simulink library "AeroModel"  (R2021b)
settings: Solver=VariableStepAuto  StartTime=0.0  StopTime=10.0  RelTol=1e-3
undefined symbols (not defined in the file or in its folder): b_ft, C_D0, C_Dalpha, C_DdeltaE, C_L0, C_Lalpha, C_Lalphadot, C_lbeta, C_ldeltaA, C_LdeltaE, C_ldeltaR, C_lp, C_Lq, C_lr, C_m0, C_malpha, C_malphadot, C_mdeltaE, C_mq, C_nbeta, C_ndeltaA, C_ndeltaR, C_np, C_nr, C_Ybeta, C_YdeltaA, C_YdeltaR, C_Yp, C_Yr, mean_c_ft, S_ft2
settings Model: Creator=setup  LastModifiedBy=dmgp1

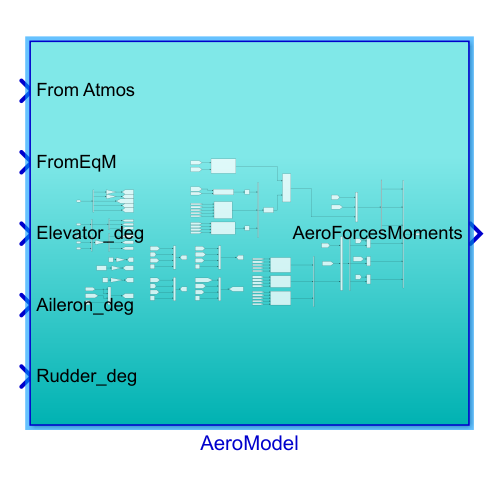
[thumbnail: Simulink's stored preview of the top-level diagram]
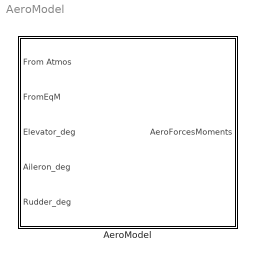
== system AeroModel ==
  AeroModel : Subsystem

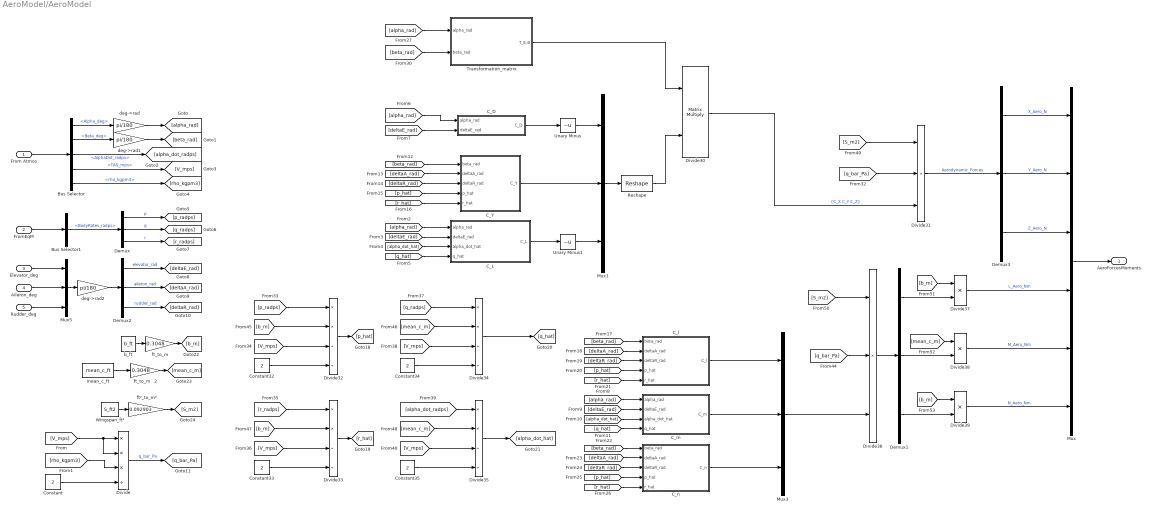
== system AeroModel/AeroModel ==
  From Atmos : Inport
  FromEqM : Inport  Port=2
  Elevator_deg : Inport  Port=3
  Aileron_deg : Inport  Port=4
  Rudder_deg : Inport  Port=5
  Bus Selector : BusSelector  OutputSignals=Alpha_deg,Beta_deg,AlphaDot_radps,TAS_mps,rho_kgpm3
  Bus Selector1 : BusSelector  OutputSignals=BodyRates_radps
  C_D : Subsystem
  C_L : Subsystem
  C_Y : Subsystem
  C_l : Subsystem
  C_m : Subsystem
  C_n : Subsystem
  Constant{,32..35} (5 alike) : Constant  Value=2
  Demux{,1..3} (4 alike) : Demux  Outputs=3
  Divide : Product  Inputs=***/
  Divide30 : Product  Inputs=**  Multiplication=Matrix(*)
  Divide31 : Product  Inputs=***
  Divide{32..35} (4 alike) : Product  Inputs=**//
  Divide36 : Product  Inputs=***
  Divide37 : Product  Inputs=**
  Divide38 : Product  Inputs=**
  Divide39 : Product  Inputs=**
  Mux : Mux  Inputs=6
  Mux1 : Mux  Inputs=3
  Mux3 : Mux  Inputs=3
  Mux5 : Mux  Inputs=3
  Reshape : Reshape  OutputDimensionality=Column vector (2-D)
  Transformation_matrix : Subsystem
  Unary Minus : UnaryMinus
  Unary Minus1 : UnaryMinus
  Wingspan_ft² : Constant  Value=S_ft2
  b_ft : Constant  Value=b_ft
  deg->rad : Gain  Gain=pi/180
  deg->rad1 : Gain  Gain=pi/180
  deg->rad2 : Gain  Gain=pi/180
  ft_to_m : Gain  Gain=0.3048
  ft_to_m   2 : Gain  Gain=0.3048
  ft²_to_m² : Gain  Gain=0.092903
  mean_c_ft : Constant  Value=mean_c_ft
  AeroForcesMoments : Outport
  wires:
  Rudder_deg/1 -> Mux5/3
  Bus Selector/3 -> [alpha_dot_radps]  "<AlphaDot_radps>"
  Bus Selector1/1 -> Demux/1  "<BodyRates_radps>"
  Demux3/3 -> Mux/3  "Z_Aero_N"
  Demux/3 -> [r_radps]  "r"
  Divide37/1 -> Mux/4  "L_Aero_Nm"
  Demux3/2 -> Mux/2  "Y_Aero_N"
  Elevator_deg/1 -> Mux5/1
  Bus Selector/5 -> [rho_kgpm3]  "<rho_kgpm3>"
  Demux/1 -> [p_radps]  "p"
  Aileron_deg/1 -> Mux5/2
  Demux/2 -> [q_radps]  "q"
  From Atmos/1 -> Bus Selector/1
  Demux3/1 -> Mux/1  "X_Aero_N"
  FromEqM/1 -> Bus Selector1/1
  Bus Selector/4 -> [V_mps]  "<TAS_mps>"
  Bus Selector/2 -> deg->rad1/1  "<Beta_deg>"
  Divide38/1 -> Mux/5  "M_Aero_Nm"
  Bus Selector/1 -> deg->rad/1  "<Alpha_deg>"
  Divide39/1 -> Mux/6  "N_Aero_Nm"
  Mux/1 -> AeroForcesMoments/1
  Constant/1 -> Divide/4
  [rho_kgpm3] -> Divide/3
  Demux1/1 -> Divide37/2
  Divide/1 -> [q_bar_Pa]  "q_bar_Pa"
  [b_m] -> Divide33/2
  [q_bar_Pa] -> Divide36/2
  Divide36/1 -> Demux1/1
  [V_mps] -> Divide32/3
  Unary Minus1/1 -> Mux1/3
  b_ft/1 -> ft_to_m/1
  [q_radps] -> Divide34/1
  Divide34/1 -> [q_hat]
  [p_radps] -> Divide32/1
  Demux1/3 -> Divide39/2
  [b_m] -> Divide37/1
  [b_m] -> Divide39/1
  [mean_c_m] -> Divide34/2
  [V_mps] -> Divide33/3
  [mean_c_m] -> Divide38/1
  [b_m] -> Divide32/2
  Demux1/2 -> Divide38/2
  [mean_c_m] -> Divide35/2
  C_m/1(C_m) -> Mux3/2
  [alpha_dot_radps] -> Divide35/1
  [S_m2] -> Divide31/1
  [V_mps] -> Divide/2, Divide/1
  Constant35/1 -> Divide35/4
  ft_to_m/1 -> [b_m]
  Mux1/1 -> Reshape/1
  Constant34/1 -> Divide34/4
  mean_c_ft/1 -> ft_to_m   2/1
  Mux3/1 -> Divide36/3
  C_l/1(C_l) -> Mux3/1
  [V_mps] -> Divide34/3
  [V_mps] -> Divide35/3
  [r_radps] -> Divide33/1
  Divide35/1 -> [alpha_dot_hat]
  C_n/1(C_n) -> Mux3/3
  Constant32/1 -> Divide32/4
  Divide33/1 -> [r_hat]
  Constant33/1 -> Divide33/4
  Divide30/1 -> Divide31/3  "{C_X C_Y C_Z}"
  [q_bar_Pa] -> Divide31/2
  Wingspan_ft²/1 -> ft²_to_m²/1
  [S_m2] -> Divide36/1
  C_D/1(C_D) -> Unary Minus/1
  Reshape/1 -> Divide30/2
  C_L/1(C_L) -> Unary Minus1/1
  ft²_to_m²/1 -> [S_m2]
  ft_to_m   2/1 -> [mean_c_m]
  C_Y/1(C_Y) -> Mux1/2
  Unary Minus/1 -> Mux1/1
  Divide32/1 -> [p_hat]
  deg->rad/1 -> [alpha_rad]
  deg->rad1/1 -> [beta_rad]
  Mux5/1 -> deg->rad2/1
  deg->rad2/1 -> Demux2/1
  Demux2/1 -> [deltaE_rad]  "elevator_rad"
  Demux2/2 -> [deltaA_rad]  "aileron_rad"
  Demux2/3 -> [deltaR_rad]  "rudder_rad"
  [alpha_rad] -> C_D/1(alpha_rad)
  [deltaE_rad] -> C_D/2(deltaE_rad)
  Transformation_matrix/1(T_E,B) -> Divide30/1
  [alpha_rad] -> Transformation_matrix/1(alpha_rad)
  [beta_rad] -> Transformation_matrix/2(beta_rad)
  [beta_rad] -> C_Y/1(beta_rad)
  [deltaA_rad] -> C_Y/2(deltaA_rad)
  [deltaR_rad] -> C_Y/3(deltaR_rad)
  [p_hat] -> C_Y/4(p_hat)
  [r_hat] -> C_Y/5(r_hat)
  [alpha_rad] -> C_L/1(alpha_rad)
  [deltaE_rad] -> C_L/2(deltaE_rad)
  [alpha_dot_hat] -> C_L/3(alpha_dot_hat)
  [q_hat] -> C_L/4(q_hat)
  Divide31/1 -> Demux3/1  "Aerodynamic_Forces"
  [beta_rad] -> C_l/1(beta_rad)
  [deltaA_rad] -> C_l/2(deltaA_rad)
  [deltaR_rad] -> C_l/3(deltaR_rad)
  [p_hat] -> C_l/4(p_hat)
  [r_hat] -> C_l/5(r_hat)
  [alpha_rad] -> C_m/1(alpha_rad)
  [deltaE_rad] -> C_m/2(deltaE_rad)
  [alpha_dot_hat] -> C_m/3(alpha_dot_hat)
  [q_hat] -> C_m/4(q_hat)
  [beta_rad] -> C_n/1(beta_rad)
  [deltaA_rad] -> C_n/2(deltaA_rad)
  [deltaR_rad] -> C_n/3(deltaR_rad)
  [p_hat] -> C_n/4(p_hat)
  [r_hat] -> C_n/5(r_hat)

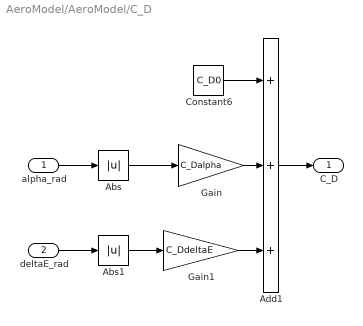
== system AeroModel/AeroModel/C_D ==
  alpha_rad : Inport
  deltaE_rad : Inport  Port=2
  Abs : Abs
  Abs1 : Abs
  Add1 : Sum  Inputs=+++
  Constant6 : Constant  Value=C_D0
  Gain : Gain  Gain=C_Dalpha
  Gain1 : Gain  Gain=C_DdeltaE
  C_D : Outport
  wires:
  Constant6/1 -> Add1/1
  deltaE_rad/1 -> Abs1/1
  Add1/1 -> C_D/1
  Abs/1 -> Gain/1
  Gain/1 -> Add1/2
  alpha_rad/1 -> Abs/1
  Gain1/1 -> Add1/3
  Abs1/1 -> Gain1/1

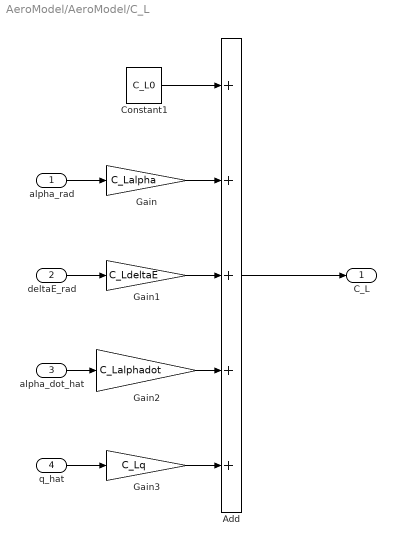
== system AeroModel/AeroModel/C_L ==
  alpha_rad : Inport
  deltaE_rad : Inport  Port=2
  alpha_dot_hat : Inport  Port=3
  q_hat : Inport  Port=4
  Add : Sum  Inputs=+++++
  Constant1 : Constant  Value=C_L0
  Gain : Gain  Gain=C_Lalpha
  Gain1 : Gain  Gain=C_LdeltaE
  Gain2 : Gain  Gain=C_Lalphadot
  Gain3 : Gain  Gain=C_Lq
  C_L : Outport
  wires:
  Gain2/1 -> Add/4
  Add/1 -> C_L/1
  Gain1/1 -> Add/3
  Gain3/1 -> Add/5
  Constant1/1 -> Add/1
  Gain/1 -> Add/2
  alpha_rad/1 -> Gain/1
  deltaE_rad/1 -> Gain1/1
  alpha_dot_hat/1 -> Gain2/1
  q_hat/1 -> Gain3/1

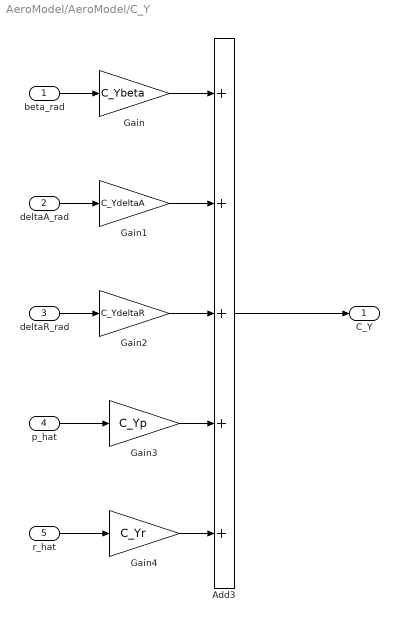
== system AeroModel/AeroModel/C_Y ==
  beta_rad : Inport
  deltaA_rad : Inport  Port=2
  deltaR_rad : Inport  Port=3
  p_hat : Inport  Port=4
  r_hat : Inport  Port=5
  Add3 : Sum  Inputs=+++++
  Gain : Gain  Gain=C_Ybeta
  Gain1 : Gain  Gain=C_YdeltaA
  Gain2 : Gain  Gain=C_YdeltaR
  Gain3 : Gain  Gain=C_Yp
  Gain4 : Gain  Gain=C_Yr
  C_Y : Outport
  wires:
  Add3/1 -> C_Y/1
  Gain1/1 -> Add3/2
  Gain/1 -> Add3/1
  Gain2/1 -> Add3/3
  Gain4/1 -> Add3/5
  Gain3/1 -> Add3/4
  beta_rad/1 -> Gain/1
  deltaA_rad/1 -> Gain1/1
  r_hat/1 -> Gain4/1
  deltaR_rad/1 -> Gain2/1
  p_hat/1 -> Gain3/1

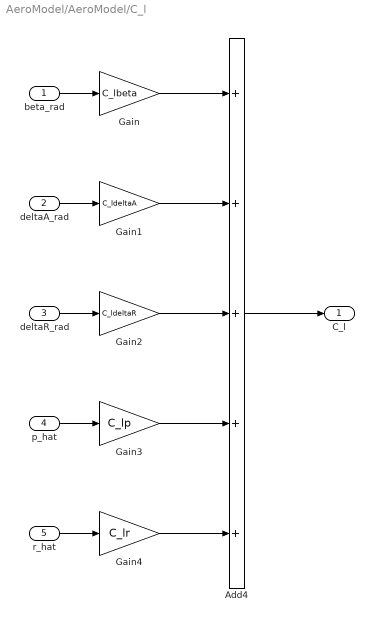
== system AeroModel/AeroModel/C_l ==
  beta_rad : Inport
  deltaA_rad : Inport  Port=2
  deltaR_rad : Inport  Port=3
  p_hat : Inport  Port=4
  r_hat : Inport  Port=5
  Add4 : Sum  Inputs=+++++
  Gain : Gain  Gain=C_lbeta
  Gain1 : Gain  Gain=C_ldeltaA
  Gain2 : Gain  Gain=C_ldeltaR
  Gain3 : Gain  Gain=C_lp
  Gain4 : Gain  Gain=C_lr
  C_l : Outport
  wires:
  Gain1/1 -> Add4/2
  Gain/1 -> Add4/1
  Add4/1 -> C_l/1
  Gain4/1 -> Add4/5
  Gain2/1 -> Add4/3
  Gain3/1 -> Add4/4
  beta_rad/1 -> Gain/1
  deltaA_rad/1 -> Gain1/1
  deltaR_rad/1 -> Gain2/1
  p_hat/1 -> Gain3/1
  r_hat/1 -> Gain4/1

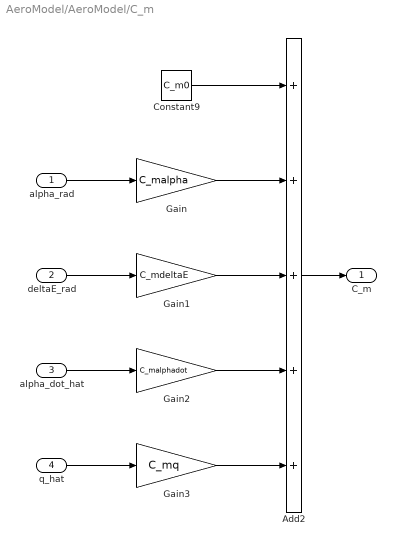
== system AeroModel/AeroModel/C_m ==
  alpha_rad : Inport
  deltaE_rad : Inport  Port=2
  alpha_dot_hat : Inport  Port=3
  q_hat : Inport  Port=4
  Add2 : Sum  Inputs=+++++
  Constant9 : Constant  Value=C_m0
  Gain : Gain  Gain=C_malpha
  Gain1 : Gain  Gain=C_mdeltaE
  Gain2 : Gain  Gain=C_malphadot
  Gain3 : Gain  Gain=C_mq
  C_m : Outport
  wires:
  Gain3/1 -> Add2/5
  Gain/1 -> Add2/2
  Add2/1 -> C_m/1
  Gain1/1 -> Add2/3
  Constant9/1 -> Add2/1
  Gain2/1 -> Add2/4
  alpha_rad/1 -> Gain/1
  deltaE_rad/1 -> Gain1/1
  alpha_dot_hat/1 -> Gain2/1
  q_hat/1 -> Gain3/1

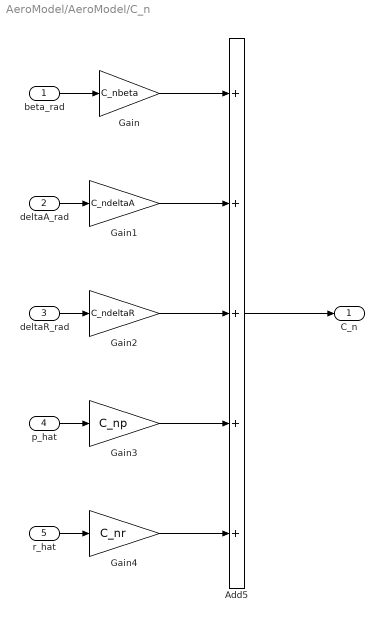
== system AeroModel/AeroModel/C_n ==
  beta_rad : Inport
  deltaA_rad : Inport  Port=2
  deltaR_rad : Inport  Port=3
  p_hat : Inport  Port=4
  r_hat : Inport  Port=5
  Add5 : Sum  Inputs=+++++
  Gain : Gain  Gain=C_nbeta
  Gain1 : Gain  Gain=C_ndeltaA
  Gain2 : Gain  Gain=C_ndeltaR
  Gain3 : Gain  Gain=C_np
  Gain4 : Gain  Gain=C_nr
  C_n : Outport
  wires:
  Gain3/1 -> Add5/4
  Gain1/1 -> Add5/2
  Add5/1 -> C_n/1
  Gain/1 -> Add5/1
  Gain2/1 -> Add5/3
  Gain4/1 -> Add5/5
  beta_rad/1 -> Gain/1
  deltaA_rad/1 -> Gain1/1
  deltaR_rad/1 -> Gain2/1
  p_hat/1 -> Gain3/1
  r_hat/1 -> Gain4/1

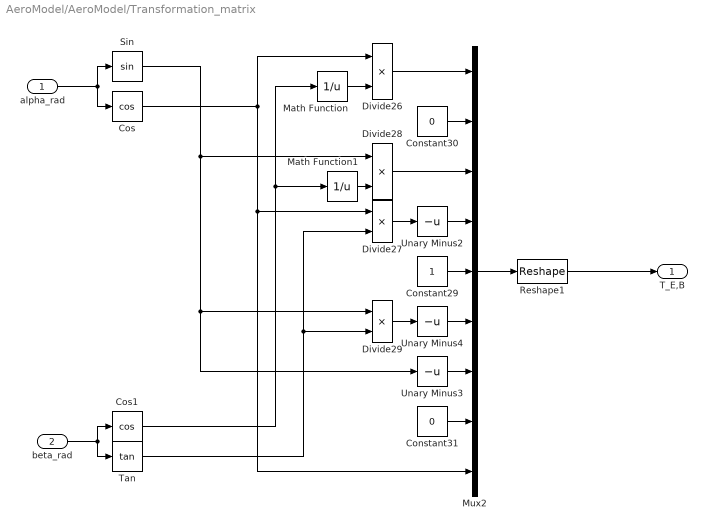
== system AeroModel/AeroModel/Transformation_matrix ==
  alpha_rad : Inport
  beta_rad : Inport  Port=2
  Constant29 : Constant
  Constant30 : Constant  Value=0
  Constant31 : Constant  Value=0
  Cos : Trigonometry  Operator=cos
  Cos1 : Trigonometry  Operator=cos
  Divide{26..29} (4 alike) : Product  Inputs=**
  Math Function : Math  Operator=reciprocal  SaturateOnIntegerOverflow=on
  Math Function1 : Math  Operator=reciprocal  SaturateOnIntegerOverflow=on
  Mux2 : Mux  Inputs=9
  Reshape1 : Reshape  OutputDimensionality=Customize  OutputDimensions=[3,3]
  Sin : Trigonometry
  Tan : Trigonometry  Operator=tan
  Unary Minus2 : UnaryMinus
  Unary Minus3 : UnaryMinus
  Unary Minus4 : UnaryMinus
  T_E,B : Outport
  wires:
  Math Function1/1 -> Divide28/2
  Sin/1 -> Divide29/1, Unary Minus3/1, Divide28/1
  Constant31/1 -> Mux2/8
  Divide26/1 -> Mux2/1
  alpha_rad/1 -> Sin/1, Cos/1
  Cos/1 -> Divide26/1, Divide27/1, Mux2/9
  Divide27/1 -> Unary Minus2/1
  Math Function/1 -> Divide26/2
  Tan/1 -> Divide27/2, Divide29/2
  Unary Minus4/1 -> Mux2/6
  Mux2/1 -> Reshape1/1
  Divide28/1 -> Mux2/3
  Divide29/1 -> Unary Minus4/1
  Cos1/1 -> Math Function1/1, Math Function/1
  Constant30/1 -> Mux2/2
  Unary Minus2/1 -> Mux2/4
  Unary Minus3/1 -> Mux2/7
  beta_rad/1 -> Tan/1, Cos1/1
  Constant29/1 -> Mux2/5
  Reshape1/1 -> T_E,B/1
